simulink model "laser_res"  (R2026a)
settings: Solver=VariableStepAuto  StopTime=7e-9  MaxStep=1e-12
values from neighbouring files (symbols this model uses):
  beta = I_0_A / (tau_sp_s * I_th_A)    [laser_tf_init.m]
  f0_sq = (I_0_A - I_th_A) / (tau_sp_s * tau_ph_s * I_th_A)    [laser_tf_init.m]
  HT_0 = ((h * c) / (lambda_m * q)) * eta_int * eta_ext * current_modifier    [laser_tf_init.m]
Description:
  | Author: Puspendu Rana
  | Project: FP Laser Simulation
  | Date: April 2026
settings Model: Creator=Puspendu Rana  LastModifiedBy=HP

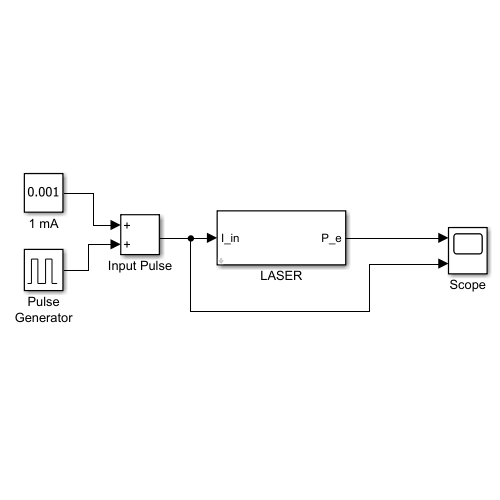
[thumbnail: Simulink's stored preview of the top-level diagram]
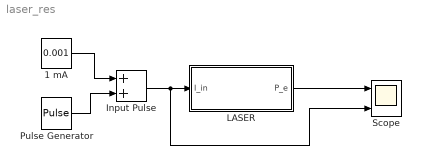
== system laser_res ==
  1 mA : Constant  Value=0.001
  Input Pulse : Sum
  LASER : Subsystem  mask(LASER MASK){tau_r=0.5, tau_nr=5, tau_ph=0.001, tau_sp=0.02, I_th=0.5, I_0=1, I_d=2, lambda=1550, L=3e-4, gamma=35e-4, R1=0.32}
      mask prompts: tau_r "Radiative recombination time (ns)"; tau_nr "Nonradiative recombination time (ns)"; tau_ph "Photon lifetime (ns)"; tau_sp "Carrier lifetime (ns)"; I_th "Threshold current (mA)"; I_0 "Pre-biasing current (mA)"; I_d "Injection current (mA)"; lambda "Emission wavelength (nm)"; L "Cavity longitudinal dimension (m)"; gamma "Loss coefficient (1/m)"; R1 "Mirror reflectancy (m)"
      mask help:
      | Fabry-Perot LASER Model
      |
      | This subsystem simulates the dynamic behaviour of a Multimode Fabry-Perot LASER diode using a small-signal frequency-domain model. It is designed to capture high-speed transient responses, including relaxation oscillations, when subjected to a modulated injection current.
      |
      | The model assumes the laser is pre-biased above its threshold current (I_d > I_th) to operate strictly within the stimulated emission region.
      |
      | The total transfer function is divided into two parts:
      | 1. DC Transfer Function (H_T(0)): Calculates the static quantum efficiency (W/A) using internal and external efficiencies.
      | 2. Dynamic Transfer Function (H_T^(s)): A 2nd-order continuous-time filter that models the photon and carrier lifetime dynamics.
      mask Help:
      | #### Overview
      | [cite_start]This block implements a linearized, small-signal model of a Fabry-Perot LASER diode suitable for high-speed telecommunication link simulations[cite: 130]. It translates frequency-domain transfer functions into standard continuous-time ($s$-domain) Simulink blocks.
      | 
      | #### Model Parameters
      | [cite_start]The simulation relies on the following physical and geometric parameters[cite: 186]:
      | 
      | | Parameter | Symbol | Description |
      | | :--- | :--- | :--- |
      | | **Emission wavelength** | $\lambda$ | Operating wavelength of the laser. |
      | | **Recombination times** | $\tau_{nr}$, $\tau_r$ | [cite_start]Non-radiative and radiative carrier lifetimes[cite: 163]. |
      | | **Cavity dimension** | $L$ | Longitudinal length of the resonant cavity. |
      | | **Loss coefficient** | $\gamma$ | Internal optical losses within the cavity. |
      | | **Mirror reflectancy** | $R_1$ | Reflectivity of the cavity facets. |
      | | **Carrier & Photon lifetimes** | $\tau_{sp}$, $\tau_{ph}$ | Time constants governing electron-hole recombination and photon decay. |
      | | **Current parameters** | $I_d$, $I_{th}$, $I_0$ | Injection, threshold, and pre-biasing currents. |
      | 
      | #### 1. Static Gain Calculation: $H_T(0)$
      | The baseline optical power efficiency is calculated as a scalar gain applied to the input current. [cite_start]It combines physical constants ($h$, $c$, $q$), the internal quantum efficiency ($\eta_{int}$), and the external quantum efficiency ($\eta_{ext}$)[cite: 160].
      | 
      | $$H_T(0) = \left( \frac{hc}{\lambda q} \right) \eta_{int} \eta_{ext} \left[ \frac{I_d - I_{th}}{I_d} \right]$$
      | 
      | [cite_start]The external quantum efficiency ($\eta_{ext}$) is derived from the cavity losses and mirror reflectance[cite: 176]:
      | 
      | $$\eta_{ext} = \frac{\ln(1/R_1)}{\gamma L + \ln(1/R_1)}$$
      | 
      | #### 2. Dynamic Transfer Function: $H_T^*(s)$
      | [cite_start]The transient response, including the characteristic ringing (relaxation oscillations) of the laser, is modeled using a normalized transfer function[cite: 177]. The frequency-domain equation is transformed into the Laplace domain ($s = j2\pi f$) for implementation in Simulink as a 2nd-order system:
      | 
      | $$H_T^*(s) = \frac{f_0^2}{s^2 + \beta s + f_0^2}$$
      | 
      | [cite_start]The resonant frequency squared ($f_0^2$) and the damping factor ($\beta$) are calculated dynamically based on the biasing conditions and carrier/photon lifetimes[cite: 178]:
      | 
      | $$f_0^2 = \frac{I_0 - I_{th}}{\tau_{sp} \tau_{ph} I_{th}}$$
      | 
      | $$\beta = \frac{I_0}{\tau_{sp} I_{th}}$$
      | 
      | #### Implementation Note
      | All mathematical constants and unit conversions (e.g., mA to A, ns to seconds) are handled automatically by the block's initialization script. [cite_start]Ensure that the input signal provided to this block includes the necessary constant DC bias ($I_0$) to maintain physical validity[cite: 187].
      mask DialogControl Container5 Prompt: Cavity & Structural Parameters
      mask DialogControl Container4 Prompt: Time Constant and Lifetimes
      mask DialogControl Container6 Prompt: Operating Currents
  Pulse Generator : DiscretePulseGenerator  PulseType=Time based  Amplitude=2e-3  Period=2e-9  PulseWidth=50
  Scope : Scope  NumInputPorts=2
      settings: Title=Input Current  ActiveDisplayYMinimum=-0.0003749999999999999  ActiveDisplayYMaximum=0.003375  YLabel=Injected Current, I_d (A)
  wires:
  LASER/1(P_e) -> Scope/1
  1 mA/1 -> Input Pulse/1
  Pulse Generator/1 -> Input Pulse/2
  Input Pulse/1 -> Scope/2, LASER/1(I_in)

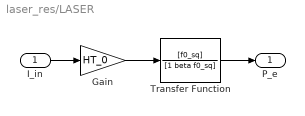
== system laser_res/LASER ==
  I_in : Inport
  Gain : Gain  Gain=HT_0
  Transfer Function : TransferFcn  Numerator=[f0_sq]  Denominator=[1 beta f0_sq]
  P_e : Outport
  wires:
  Transfer Function/1 -> P_e/1
  I_in/1 -> Gain/1
  Gain/1 -> Transfer Function/1
